simulink model "Consensus_Swarm"  (R2023b)
settings: Solver=ode3  StartTime=0.0  StopTime=inf  FixedStep=0.001  RelTol=1e-3
values from neighbouring files (symbols this model uses):
  g = 9.8    [Parameters.m]
  Ic = [2 0 0; 0 2 0; 0 0 4]    [Parameters.m]
  m = 1    [Parameters.m]
  M_RB = [eye(3), zeros(3); zeros(3), I]    [Parameters.m]
  SAVE_SPACE = 5    [Parameters.m]
  STEP_SIZE = 1    [Parameters.m]
libraries: simulink_extras x36, slpidlib x36, aerolibutil x12, vrlib x7
(part 6 of 6)

== system Consensus_Swarm/Subsystem/LIDER/Quadcopter model/Rigid-body dynamics ==
  note: $\nu$
  tau_g : Inport
  tau_p : Inport  Port=2
  Constant : Constant  Value=m
  Constant1 : Constant  Value=Ic  VectorParams1D=off
  Coriolis term : MATLAB Function  TreatAsAtomicUnit=on
  Gain : Gain  Gain=inv(M_RB)  Multiplication=Matrix(K*u) (u vector)
  Integrator1 : Integrator  InitialCondition=[0;0;0;0;0;0]
  Sum : Sum  Inputs=++-
  nu : Outport
  wires:
  Integrator1/1 -> nu/1, Coriolis term/1(nu)
  Constant/1 -> Coriolis term/2(m)
  Sum/1 -> Gain/1
  tau_p/1 -> Sum/2
  Coriolis term/1(Cnunu) -> Sum/3
  Constant1/1 -> Coriolis term/3(Ic)
  Gain/1 -> Integrator1/1
  tau_g/1 -> Sum/1

== system Consensus_Swarm/Subsystem/LIDER/Quadcopter model/gravity ==
  R_be : Inport
  Manual Switch : ManualSwitch
  Math Function : Math  Operator=transpose
  Matrix Multiply : Product  Multiplication=Matrix(*)
  Mux2 : Mux  Inputs=2
  gravity vector : Constant  Value=[0;0;m*g]  VectorParams1D=off
  zeros : Constant  Value=[0;0;0]  VectorParams1D=off
  tau_g : Outport
  wires:
  Matrix Multiply/1 -> Manual Switch/1
  Manual Switch/1 -> Mux2/1
  Mux2/1 -> tau_g/1
  gravity vector/1 -> Matrix Multiply/2
  zeros/1 -> Mux2/2, Manual Switch/2
  Math Function/1 -> Matrix Multiply/1
  R_be/1 -> Math Function/1

== matlab function Consensus_Swarm/MATLAB Function1 ==
  data: p1 input; all_pose output; p2 input; p3 input; p4 input; p5 input; p6 input
function all_pose = Format(p1,p2,p3,p4,p5,p6)

%y = [p1';p2';p3';p4']';
all_pose = [p1';p2';p3';p4';p5';p6'];

== matlab function Consensus_Swarm/FOLLOWER 2/Agent Model/Flight Control System/Outer loop position control/MATLAB Function ==
  data: Deltap_e input; Deltap_b output; psi input
function Deltap_b = fcn(Deltap_e,psi)

R = [ cos(psi) , -sin(psi) ;
      sin(psi) ,  cos(psi) ];

Deltap_b = R'*Deltap_e;

== matlab function Consensus_Swarm/FOLLOWER 2/Agent Model/Quadcopter model/Kinematics/Kinematics ==
  data: R_be output; nu input; eta input; eta_dot output
function [R_be,eta_dot] = J_Theta(nu,eta)

% Euler angle extraction
phi = eta(4);
theta = eta(5);
psi = eta(6);

R_xphi = [ 1 0 0 ; 0 cos(phi) -sin(phi) ; 0 sin(phi) cos(phi) ];
R_ytheta = [ cos(theta) 0 sin(theta) ; 0 1 0 ; -sin(theta) 0 cos(theta) ];
R_zpsi = [ cos(psi) -sin(psi) 0 ; sin(psi) cos(psi) 0 ; 0 0 1 ];

% rotation matrix
R_be = R_zpsi * R_ytheta * R_xphi;

% angular velocity transformation
T_Theta = [ 1 sin(phi)*tan(theta) cos(phi)*tan(theta) ; 0 cos(phi) -sin(phi) ; 0 sin(phi)/cos(theta) cos(phi)/cos(theta) ];

J_Theta = [ R_be , zeros(3) ; zeros(3) , T_Theta ];

eta_dot = J_Theta*nu;

== matlab function Consensus_Swarm/gamepad/Formatting/MATLAB Function ==
  data: L1 input; y output; R1 input
function y = fcn(L1, R1)

if L1 == 1 && R1 == 0
    y = -1;
elseif R1 == 1 && L1 == 0
    y = 1;
else
    y = 0;
end

end

== matlab function Consensus_Swarm/FOLLOWER 3/MATLAB Function1 ==
  data: id input; others input; base_speed input; ref output
function ref = Aggregation(id, others, base_speed)

% Get self position based on individual ID:
self_pose = others(id,:);


% Compute distance difference:
adjustment = [0,0,0,0];

for i = 1:length(others)
    other_pose = others(i,:);

    adjustment = adjustment + (other_pose - self_pose);

end
   
ref = self_pose + base_speed*adjustment;

end

== matlab function Consensus_Swarm/FOLLOWER 2/Agent Model/Quadcopter model/Rigid-body dynamics/Coriolis term ==
  data: nu input; Cnunu output; m input; Ic input
function Cnunu = fcn(nu,m,Ic)

v = nu(1:3);  % linear velocities (expressed in the body frame)
omega = nu(4:6); % angular velocities (expressed in the body frame)


Cnunu = [ cross(omega,m*v) ; -cross(Ic*omega,omega) ];

== matlab function Consensus_Swarm/FOLLOWER 2/MATLAB Function ==
  data: id input; others input; base_speed input; ref output; d input; angle output
function [ref, angle] = Chain(id, others, base_speed, d)

% Get self position based on individual ID:
self_pose = others(id,:);

 % Get Lider position (always ID 1)
lider_pose = others(id-1,:);

% Compute offset:
angle = lider_pose(4);
offset = [cos(angle)*d, sin(angle)*d, 0, 0];

delta = lider_pose - offset - self_pose;


new_pose = self_pose + base_speed*delta;

% Modify control input:
new_x = new_pose(1);
new_y = new_pose(2);
new_z = new_pose(3);
new_psi = new_pose(4);

ref = [new_x;new_y;new_z;new_psi];

end

== matlab function Consensus_Swarm/FOLLOWER 2/MATLAB Function1 ==
  data: id input; others input; base_speed input; ref output
function ref = Aggregation(id, others, base_speed)

% Get self position based on individual ID:
self_pose = others(id,:);


% Compute distance difference:
adjustment = [0,0,0,0];

for i = 1:length(others)
    other_pose = others(i,:);

    adjustment = adjustment + (other_pose - self_pose);

end
   
ref = self_pose + base_speed*adjustment;

end

== matlab function Consensus_Swarm/FOLLOWER 2/MATLAB Function10 ==
  data: id input; new_ref output; ref input; others input; safe_space input
function new_ref = AvoidCollision(id, ref, others, safe_space)
    
% Extract control input:
new_x = ref(1);
new_y = ref(2);
new_z = ref(3);
new_psi = ref(4);

% Get self position based on individual ID:
self_pose = others(id,1:3);
x = self_pose(1);
y = self_pose(2);
z = self_pose(3);

% Position difference:
adjustment = [0,0,0];
for i = 1:length(others)
    n_x = others(i, 1);
    n_y = others(i, 2);
    n_z = others(i, 3);
    
    if i ~= id   % Not take self position twice
        % Compute distance:
        distance = sqrt((x - n_x)^2 + (y - n_y)^2 + (z - n_z)^2);
        
        if distance < safe_space
            % Compute adjustment vector:
            adjustment = [(x - n_x), (y - n_y), (z - n_z)];
            adjustment = adjustment/distance;
            adjustment = adjustment*((safe_space - distance)/2);
    
            % Modify control input:
            new_x = new_x + adjustment(1);
            new_y = new_y + adjustment(2);
            new_z = new_z + adjustment(3);
        end
    end
    new_ref = [new_x;new_y;new_z;new_psi];
end

== matlab function Consensus_Swarm/gamepad/MATLAB Function7 ==
  data: scale_factor input; d_new output; angle_factor input; d input; phi input; phi_new output
function [d_new, phi_new]= fcn(scale_factor, angle_factor, d, phi)

d_new = d + scale_factor;


phi_new = phi + angle_factor;

if phi_new > 2*pi
    phi_new = phi_new - 2*pi;
elseif phi_new < -2*pi
    phi_new = phi_new + 2*pi;
end

== matlab function Consensus_Swarm/FOLLOWER 2/MATLAB Function11 ==
  data: id input; ref output; others input; d input; phi input; base_speed input
function ref = ShapeForming(id, others, d, phi, base_speed)

% Get self position based on individual ID:
self_pose = others(id,:);

% Get Lider position (always ID 1)
lider_pose = others(1,:);

% Number of drones:
drone_number = length(others);

% Compute offset:
angle = phi  + id*(2*pi/(drone_number-1));
offset = [d*cos(angle), d*sin(angle), 0, 0];

delta = lider_pose - offset - self_pose;

new_pose = self_pose + base_speed*delta;

% Modify control input:
new_x = new_pose(1);
new_y = new_pose(2);
new_z = new_pose(3);
new_psi = new_pose(4);

ref = [new_x;new_y;new_z;new_psi];

== matlab function Consensus_Swarm/FOLLOWER 3/Agent Model/Flight Control System/Outer loop position control/MATLAB Function ==
  data: Deltap_e input; Deltap_b output; psi input
function Deltap_b = fcn(Deltap_e,psi)

R = [ cos(psi) , -sin(psi) ;
      sin(psi) ,  cos(psi) ];

Deltap_b = R'*Deltap_e;

== matlab function Consensus_Swarm/FOLLOWER 3/Agent Model/Quadcopter model/Kinematics/Kinematics ==
  data: R_be output; nu input; eta input; eta_dot output
function [R_be,eta_dot] = J_Theta(nu,eta)

% Euler angle extraction
phi = eta(4);
theta = eta(5);
psi = eta(6);

R_xphi = [ 1 0 0 ; 0 cos(phi) -sin(phi) ; 0 sin(phi) cos(phi) ];
R_ytheta = [ cos(theta) 0 sin(theta) ; 0 1 0 ; -sin(theta) 0 cos(theta) ];
R_zpsi = [ cos(psi) -sin(psi) 0 ; sin(psi) cos(psi) 0 ; 0 0 1 ];

% rotation matrix
R_be = R_zpsi * R_ytheta * R_xphi;

% angular velocity transformation
T_Theta = [ 1 sin(phi)*tan(theta) cos(phi)*tan(theta) ; 0 cos(phi) -sin(phi) ; 0 sin(phi)/cos(theta) cos(phi)/cos(theta) ];

J_Theta = [ R_be , zeros(3) ; zeros(3) , T_Theta ];

eta_dot = J_Theta*nu;

== matlab function Consensus_Swarm/FOLLOWER 3/Agent Model/Quadcopter model/Rigid-body dynamics/Coriolis term ==
  data: nu input; Cnunu output; m input; Ic input
function Cnunu = fcn(nu,m,Ic)

v = nu(1:3);  % linear velocities (expressed in the body frame)
omega = nu(4:6); % angular velocities (expressed in the body frame)


Cnunu = [ cross(omega,m*v) ; -cross(Ic*omega,omega) ];

== matlab function Consensus_Swarm/FOLLOWER 3/MATLAB Function ==
  data: id input; others input; base_speed input; ref output; d input; angle output
function [ref, angle] = Chain(id, others, base_speed, d)

% Get self position based on individual ID:
self_pose = others(id,:);

 % Get Lider position (always ID 1)
lider_pose = others(id-1,:);

% Compute offset:
angle = lider_pose(4);
offset = [cos(angle)*d, sin(angle)*d, 0, 0];

delta = lider_pose - offset - self_pose;


new_pose = self_pose + base_speed*delta;

% Modify control input:
new_x = new_pose(1);
new_y = new_pose(2);
new_z = new_pose(3);
new_psi = new_pose(4);

ref = [new_x;new_y;new_z;new_psi];

end

== matlab function Consensus_Swarm/FOLLOWER 3/MATLAB Function10 ==
  data: id input; new_ref output; ref input; others input; safe_space input
function new_ref = AvoidCollision(id, ref, others, safe_space)
    
% Extract control input:
new_x = ref(1);
new_y = ref(2);
new_z = ref(3);
new_psi = ref(4);

% Get self position based on individual ID:
self_pose = others(id,1:3);
x = self_pose(1);
y = self_pose(2);
z = self_pose(3);

% Position difference:
adjustment = [0,0,0];
for i = 1:length(others)
    n_x = others(i, 1);
    n_y = others(i, 2);
    n_z = others(i, 3);
    
    if i ~= id   % Not take self position twice
        % Compute distance:
        distance = sqrt((x - n_x)^2 + (y - n_y)^2 + (z - n_z)^2);
        
        if distance < safe_space
            % Compute adjustment vector:
            adjustment = [(x - n_x), (y - n_y), (z - n_z)];
            adjustment = adjustment/distance;
            adjustment = adjustment*((safe_space - distance)/2);
    
            % Modify control input:
            new_x = new_x + adjustment(1);
            new_y = new_y + adjustment(2);
            new_z = new_z + adjustment(3);
        end
    end
    new_ref = [new_x;new_y;new_z;new_psi];
end

== matlab function Consensus_Swarm/FOLLOWER 3/MATLAB Function11 ==
  data: id input; ref output; others input; d input; phi input; base_speed input
function ref = ShapeForming(id, others, d, phi, base_speed)

% Get self position based on individual ID:
self_pose = others(id,:);

% Get Lider position (always ID 1)
lider_pose = others(1,:);

% Number of drones:
drone_number = length(others);

% Compute offset:
angle = phi  + id*(2*pi/(drone_number-1));
offset = [d*cos(angle), d*sin(angle), 0, 0];

delta = lider_pose - offset - self_pose;

new_pose = self_pose + base_speed*delta;

% Modify control input:
new_x = new_pose(1);
new_y = new_pose(2);
new_z = new_pose(3);
new_psi = new_pose(4);

ref = [new_x;new_y;new_z;new_psi];

== matlab function Consensus_Swarm/Subsystem/LIDER/Flight Control System/Outer loop position control/MATLAB Function ==
  data: Deltap_e input; Deltap_b output; psi input
function Deltap_b = fcn(Deltap_e,psi)

R = [ cos(psi) , -sin(psi) ;
      sin(psi) ,  cos(psi) ];

Deltap_b = R'*Deltap_e;

== matlab function Consensus_Swarm/Subsystem/LIDER/Quadcopter model/Kinematics/Kinematics ==
  data: R_be output; nu input; eta input; eta_dot output
function [R_be,eta_dot] = J_Theta(nu,eta)

% Euler angle extraction
phi = eta(4);
theta = eta(5);
psi = eta(6);

R_xphi = [ 1 0 0 ; 0 cos(phi) -sin(phi) ; 0 sin(phi) cos(phi) ];
R_ytheta = [ cos(theta) 0 sin(theta) ; 0 1 0 ; -sin(theta) 0 cos(theta) ];
R_zpsi = [ cos(psi) -sin(psi) 0 ; sin(psi) cos(psi) 0 ; 0 0 1 ];

% rotation matrix
R_be = R_zpsi * R_ytheta * R_xphi;

% angular velocity transformation
T_Theta = [ 1 sin(phi)*tan(theta) cos(phi)*tan(theta) ; 0 cos(phi) -sin(phi) ; 0 sin(phi)/cos(theta) cos(phi)/cos(theta) ];

J_Theta = [ R_be , zeros(3) ; zeros(3) , T_Theta ];

eta_dot = J_Theta*nu;

== matlab function Consensus_Swarm/Subsystem/LIDER/Quadcopter model/Rigid-body dynamics/Coriolis term ==
  data: nu input; Cnunu output; m input; Ic input
function Cnunu = fcn(nu,m,Ic)

v = nu(1:3);  % linear velocities (expressed in the body frame)
omega = nu(4:6); % angular velocities (expressed in the body frame)


Cnunu = [ cross(omega,m*v) ; -cross(Ic*omega,omega) ];

== matlab function Consensus_Swarm/gamepad/MATLAB Function ==
  data: x input; new_mode output; circle input; square input; mode input
function new_mode = SelectMode(x,circle,square, mode)

new_mode = mode
if x == 1
    new_mode = 3;
elseif circle == 1
    new_mode = 1;
elseif square == 1
    new_mode = 2;

end
end

== matlab function Consensus_Swarm/FOLLOWER 4/Agent Model/Flight Control System/Outer loop position control/MATLAB Function ==
  data: Deltap_e input; Deltap_b output; psi input
function Deltap_b = fcn(Deltap_e,psi)

R = [ cos(psi) , -sin(psi) ;
      sin(psi) ,  cos(psi) ];

Deltap_b = R'*Deltap_e;

== matlab function Consensus_Swarm/FOLLOWER 4/Agent Model/Quadcopter model/Kinematics/Kinematics ==
  data: R_be output; nu input; eta input; eta_dot output
function [R_be,eta_dot] = J_Theta(nu,eta)

% Euler angle extraction
phi = eta(4);
theta = eta(5);
psi = eta(6);

R_xphi = [ 1 0 0 ; 0 cos(phi) -sin(phi) ; 0 sin(phi) cos(phi) ];
R_ytheta = [ cos(theta) 0 sin(theta) ; 0 1 0 ; -sin(theta) 0 cos(theta) ];
R_zpsi = [ cos(psi) -sin(psi) 0 ; sin(psi) cos(psi) 0 ; 0 0 1 ];

% rotation matrix
R_be = R_zpsi * R_ytheta * R_xphi;

% angular velocity transformation
T_Theta = [ 1 sin(phi)*tan(theta) cos(phi)*tan(theta) ; 0 cos(phi) -sin(phi) ; 0 sin(phi)/cos(theta) cos(phi)/cos(theta) ];

J_Theta = [ R_be , zeros(3) ; zeros(3) , T_Theta ];

eta_dot = J_Theta*nu;

== matlab function Consensus_Swarm/FOLLOWER 4/Agent Model/Quadcopter model/Rigid-body dynamics/Coriolis term ==
  data: nu input; Cnunu output; m input; Ic input
function Cnunu = fcn(nu,m,Ic)

v = nu(1:3);  % linear velocities (expressed in the body frame)
omega = nu(4:6); % angular velocities (expressed in the body frame)


Cnunu = [ cross(omega,m*v) ; -cross(Ic*omega,omega) ];

== matlab function Consensus_Swarm/FOLLOWER 4/MATLAB Function ==
  data: id input; others input; base_speed input; ref output; d input; angle output
function [ref, angle] = Chain(id, others, base_speed, d)

% Get self position based on individual ID:
self_pose = others(id,:);

 % Get Lider position (always ID 1)
lider_pose = others(id-1,:);

% Compute offset:
angle = lider_pose(4);
offset = [cos(angle)*d, sin(angle)*d, 0, 0];

delta = lider_pose - offset - self_pose;


new_pose = self_pose + base_speed*delta;

% Modify control input:
new_x = new_pose(1);
new_y = new_pose(2);
new_z = new_pose(3);
new_psi = new_pose(4);

ref = [new_x;new_y;new_z;new_psi];

end

== matlab function Consensus_Swarm/FOLLOWER 4/MATLAB Function1 ==
  data: id input; others input; base_speed input; ref output
function ref = Aggregation(id, others, base_speed)

% Get self position based on individual ID:
self_pose = others(id,:);


% Compute distance difference:
adjustment = [0,0,0,0];

for i = 1:length(others)
    other_pose = others(i,:);

    adjustment = adjustment + (other_pose - self_pose);

end
   
ref = self_pose + base_speed*adjustment;

end

== matlab function Consensus_Swarm/FOLLOWER 4/MATLAB Function10 ==
  data: id input; new_ref output; ref input; others input; safe_space input
function new_ref = AvoidCollision(id, ref, others, safe_space)
    
% Extract control input:
new_x = ref(1);
new_y = ref(2);
new_z = ref(3);
new_psi = ref(4);

% Get self position based on individual ID:
self_pose = others(id,1:3);
x = self_pose(1);
y = self_pose(2);
z = self_pose(3);

% Position difference:
adjustment = [0,0,0];
for i = 1:length(others)
    n_x = others(i, 1);
    n_y = others(i, 2);
    n_z = others(i, 3);
    
    if i ~= id   % Not take self position twice
        % Compute distance:
        distance = sqrt((x - n_x)^2 + (y - n_y)^2 + (z - n_z)^2);
        
        if distance < safe_space
            % Compute adjustment vector:
            adjustment = [(x - n_x), (y - n_y), (z - n_z)];
            adjustment = adjustment/distance;
            adjustment = adjustment*((safe_space - distance)/2);
    
            % Modify control input:
            new_x = new_x + adjustment(1);
            new_y = new_y + adjustment(2);
            new_z = new_z + adjustment(3);
        end
    end
    new_ref = [new_x;new_y;new_z;new_psi];
end

== matlab function Consensus_Swarm/FOLLOWER 1/Agent Model/Flight Control System/Outer loop position control/MATLAB Function ==
  data: Deltap_e input; Deltap_b output; psi input
function Deltap_b = fcn(Deltap_e,psi)

R = [ cos(psi) , -sin(psi) ;
      sin(psi) ,  cos(psi) ];

Deltap_b = R'*Deltap_e;

== matlab function Consensus_Swarm/FOLLOWER 4/MATLAB Function11 ==
  data: id input; ref output; others input; d input; phi input; base_speed input
function ref = ShapeForming(id, others, d, phi, base_speed)

% Get self position based on individual ID:
self_pose = others(id,:);

% Get Lider position (always ID 1)
lider_pose = others(1,:);

% Number of drones:
drone_number = length(others);

% Compute offset:
angle = phi  + id*(2*pi/(drone_number-1));
offset = [d*cos(angle), d*sin(angle), 0, 0];

delta = lider_pose - offset - self_pose;

new_pose = self_pose + base_speed*delta;

% Modify control input:
new_x = new_pose(1);
new_y = new_pose(2);
new_z = new_pose(3);
new_psi = new_pose(4);

ref = [new_x;new_y;new_z;new_psi];

== matlab function Consensus_Swarm/FOLLOWER 5/Agent Model/Flight Control System/Outer loop position control/MATLAB Function ==
  data: Deltap_e input; Deltap_b output; psi input
function Deltap_b = fcn(Deltap_e,psi)

R = [ cos(psi) , -sin(psi) ;
      sin(psi) ,  cos(psi) ];

Deltap_b = R'*Deltap_e;

== matlab function Consensus_Swarm/FOLLOWER 5/Agent Model/Quadcopter model/Kinematics/Kinematics ==
  data: R_be output; nu input; eta input; eta_dot output
function [R_be,eta_dot] = J_Theta(nu,eta)

% Euler angle extraction
phi = eta(4);
theta = eta(5);
psi = eta(6);

R_xphi = [ 1 0 0 ; 0 cos(phi) -sin(phi) ; 0 sin(phi) cos(phi) ];
R_ytheta = [ cos(theta) 0 sin(theta) ; 0 1 0 ; -sin(theta) 0 cos(theta) ];
R_zpsi = [ cos(psi) -sin(psi) 0 ; sin(psi) cos(psi) 0 ; 0 0 1 ];

% rotation matrix
R_be = R_zpsi * R_ytheta * R_xphi;

% angular velocity transformation
T_Theta = [ 1 sin(phi)*tan(theta) cos(phi)*tan(theta) ; 0 cos(phi) -sin(phi) ; 0 sin(phi)/cos(theta) cos(phi)/cos(theta) ];

J_Theta = [ R_be , zeros(3) ; zeros(3) , T_Theta ];

eta_dot = J_Theta*nu;

== matlab function Consensus_Swarm/FOLLOWER 5/Agent Model/Quadcopter model/Rigid-body dynamics/Coriolis term ==
  data: nu input; Cnunu output; m input; Ic input
function Cnunu = fcn(nu,m,Ic)

v = nu(1:3);  % linear velocities (expressed in the body frame)
omega = nu(4:6); % angular velocities (expressed in the body frame)


Cnunu = [ cross(omega,m*v) ; -cross(Ic*omega,omega) ];

== matlab function Consensus_Swarm/FOLLOWER 5/MATLAB Function ==
  data: id input; others input; base_speed input; ref output; d input; angle output
function [ref, angle] = Chain(id, others, base_speed, d)

% Get self position based on individual ID:
self_pose = others(id,:);

 % Get Lider position (always ID 1)
lider_pose = others(id-1,:);

% Compute offset:
angle = lider_pose(4);
offset = [cos(angle)*d, sin(angle)*d, 0, 0];

delta = lider_pose - offset - self_pose;


new_pose = self_pose + base_speed*delta;

% Modify control input:
new_x = new_pose(1);
new_y = new_pose(2);
new_z = new_pose(3);
new_psi = new_pose(4);

ref = [new_x;new_y;new_z;new_psi];

end

== matlab function Consensus_Swarm/FOLLOWER 5/MATLAB Function1 ==
  data: id input; others input; base_speed input; ref output
function ref = Aggregation(id, others, base_speed)

% Get self position based on individual ID:
self_pose = others(id,:);


% Compute distance difference:
adjustment = [0,0,0,0];

for i = 1:length(others)
    other_pose = others(i,:);

    adjustment = adjustment + (other_pose - self_pose);

end
   
ref = self_pose + base_speed*adjustment;

end

== matlab function Consensus_Swarm/FOLLOWER 5/MATLAB Function10 ==
  data: id input; new_ref output; ref input; others input; safe_space input
function new_ref = AvoidCollision(id, ref, others, safe_space)
    
% Extract control input:
new_x = ref(1);
new_y = ref(2);
new_z = ref(3);
new_psi = ref(4);

% Get self position based on individual ID:
self_pose = others(id,1:3);
x = self_pose(1);
y = self_pose(2);
z = self_pose(3);

% Position difference:
adjustment = [0,0,0];
for i = 1:length(others)
    n_x = others(i, 1);
    n_y = others(i, 2);
    n_z = others(i, 3);
    
    if i ~= id   % Not take self position twice
        % Compute distance:
        distance = sqrt((x - n_x)^2 + (y - n_y)^2 + (z - n_z)^2);
        
        if distance < safe_space
            % Compute adjustment vector:
            adjustment = [(x - n_x), (y - n_y), (z - n_z)];
            adjustment = adjustment/distance;
            adjustment = adjustment*((safe_space - distance)/2);
    
            % Modify control input:
            new_x = new_x + adjustment(1);
            new_y = new_y + adjustment(2);
            new_z = new_z + adjustment(3);
        end
    end
    new_ref = [new_x;new_y;new_z;new_psi];
end

== matlab function Consensus_Swarm/FOLLOWER 5/MATLAB Function11 ==
  data: id input; ref output; others input; d input; phi input; base_speed input
function ref = ShapeForming(id, others, d, phi, base_speed)

% Get self position based on individual ID:
self_pose = others(id,:);

% Get Lider position (always ID 1)
lider_pose = others(1,:);

% Number of drones:
drone_number = length(others);

% Compute offset:
angle = phi  + id*(2*pi/(drone_number-1));
offset = [d*cos(angle), d*sin(angle), 0, 0];

delta = lider_pose - offset - self_pose;

new_pose = self_pose + base_speed*delta;

% Modify control input:
new_x = new_pose(1);
new_y = new_pose(2);
new_z = new_pose(3);
new_psi = new_pose(4);

ref = [new_x;new_y;new_z;new_psi];

== matlab function Consensus_Swarm/FOLLOWER 1/Agent Model/Quadcopter model/Kinematics/Kinematics ==
  data: R_be output; nu input; eta input; eta_dot output
function [R_be,eta_dot] = J_Theta(nu,eta)

% Euler angle extraction
phi = eta(4);
theta = eta(5);
psi = eta(6);

R_xphi = [ 1 0 0 ; 0 cos(phi) -sin(phi) ; 0 sin(phi) cos(phi) ];
R_ytheta = [ cos(theta) 0 sin(theta) ; 0 1 0 ; -sin(theta) 0 cos(theta) ];
R_zpsi = [ cos(psi) -sin(psi) 0 ; sin(psi) cos(psi) 0 ; 0 0 1 ];

% rotation matrix
R_be = R_zpsi * R_ytheta * R_xphi;

% angular velocity transformation
T_Theta = [ 1 sin(phi)*tan(theta) cos(phi)*tan(theta) ; 0 cos(phi) -sin(phi) ; 0 sin(phi)/cos(theta) cos(phi)/cos(theta) ];

J_Theta = [ R_be , zeros(3) ; zeros(3) , T_Theta ];

eta_dot = J_Theta*nu;

== matlab function Consensus_Swarm/FOLLOWER 1/Agent Model/Quadcopter model/Rigid-body dynamics/Coriolis term ==
  data: nu input; Cnunu output; m input; Ic input
function Cnunu = fcn(nu,m,Ic)

v = nu(1:3);  % linear velocities (expressed in the body frame)
omega = nu(4:6); % angular velocities (expressed in the body frame)


Cnunu = [ cross(omega,m*v) ; -cross(Ic*omega,omega) ];

== matlab function Consensus_Swarm/FOLLOWER 1/MATLAB Function ==
  data: id input; others input; base_speed input; ref output; d input; angle output
function [ref, angle] = Chain(id, others, base_speed, d)

% Get self position based on individual ID:
self_pose = others(id,:);

 % Get Lider position (always ID 1)
lider_pose = others(id-1,:);

% Compute offset:
angle = lider_pose(4);
offset = [cos(angle)*d, sin(angle)*d, 0, 0];

delta = lider_pose - offset - self_pose;


new_pose = self_pose + base_speed*delta;

% Modify control input:
new_x = new_pose(1);
new_y = new_pose(2);
new_z = new_pose(3);
new_psi = new_pose(4);

ref = [new_x;new_y;new_z;new_psi];

end

== matlab function Consensus_Swarm/FOLLOWER 1/MATLAB Function1 ==
  data: id input; others input; base_speed input; ref output
function ref = Aggregation(id, others, base_speed)

% Get self position based on individual ID:
self_pose = others(id,:);


% Compute distance difference:
adjustment = [0,0,0,0];

for i = 1:length(others)
    other_pose = others(i,:);

    adjustment = adjustment + (other_pose - self_pose);

end
   
ref = self_pose + base_speed*adjustment;

end

== matlab function Consensus_Swarm/FOLLOWER 1/MATLAB Function10 ==
  data: id input; new_ref output; ref input; others input; safe_space input
function new_ref = AvoidCollision(id, ref, others, safe_space)
    
% Extract control input:
new_x = ref(1);
new_y = ref(2);
new_z = ref(3);
new_psi = ref(4);

% Get self position based on individual ID:
self_pose = others(id,1:3);
x = self_pose(1);
y = self_pose(2);
z = self_pose(3);

% Position difference:
adjustment = [0,0,0];
for i = 1:length(others)
    n_x = others(i, 1);
    n_y = others(i, 2);
    n_z = others(i, 3);
    
    if i ~= id   % Not take self position twice
        % Compute distance:
        distance = sqrt((x - n_x)^2 + (y - n_y)^2 + (z - n_z)^2);
        
        if distance < safe_space
            % Compute adjustment vector:
            adjustment = [(x - n_x), (y - n_y), (z - n_z)];
            adjustment = adjustment/distance;
            adjustment = adjustment*((safe_space - distance)/2);
    
            % Modify control input:
            new_x = new_x + adjustment(1);
            new_y = new_y + adjustment(2);
            new_z = new_z + adjustment(3);
        end
    end
    new_ref = [new_x;new_y;new_z;new_psi];
end

== matlab function Consensus_Swarm/FOLLOWER 1/MATLAB Function11 ==
  data: id input; ref output; others input; d input; phi input; base_speed input
function ref = ShapeForming(id, others, d, phi, base_speed)

% Get self position based on individual ID:
self_pose = others(id,:);

% Get Lider position (always ID 1)
lider_pose = others(1,:);

% Number of drones:
drone_number = length(others);

% Compute offset:
angle = phi  + id*(2*pi/(drone_number-1));
offset = [d*cos(angle), d*sin(angle), 0, 0];

delta = lider_pose - offset - self_pose;


new_pose = self_pose + base_speed*delta;

% Modify control input:
new_x = new_pose(1);
new_y = new_pose(2);
new_z = new_pose(3);
new_psi = new_pose(4);

ref = [new_x;new_y;new_z;new_psi];
